simulink model "CalibrationMotorbike_v2"  (R2020b)
settings: Solver=FixedStepDiscrete  StartTime=0.0  StopTime=inf  FixedStep=0.01  RelTol=1e-3  EnableMultiTasking=on
undefined symbols (not defined in the file or in its folder): fdesignblkfcn, gcbh
libraries: dspstat3 x11, dsparch4 x3, simulink x2, dspswit3 x1
(part 1 of 2)
settings Model: DataDictionary=MOCA_DD.sldd  EnableAccessToBaseWorkspace=off  DataTypeOverride=Off  DataTypeOverrideAppliesTo=Floating-point  MinMaxOverflowLogging=ForceOff  SimulationMode=accelerator  OrderedModelArguments=off  Creator=stj1si  LastModifiedBy=HNA3SI
settings DataIOCC: SaveFormat=Array  SaveOutput=off  SignalLogging=off  SaveTime=off  ReturnWorkspaceOutputs=off
settings OptimizationCC: DefaultParameterBehavior=Inlined  DefaultUnderspecifiedDataType=single  InlineInvariantSignals=on  EnhancedBackFolding=on  CachingGlobalReferences=on  ExpressionDepthLimit=2147483647  NoFixptDivByZeroProtection=on  EfficientFloat2IntCast=on  LifeSpan=1  SimCompilerOptimization=on  EfficientTunableParamExpr=on
settings DebuggingCC: SolverPrmCheckMsg=warning  ParameterPrecisionLossMsg=none  AllowSymbolicDim=off  StateNameClashWarn=warning  SFUnexpectedBacktrackingDiag=warning  SFNoUnconditionalDefaultTransitionDiag=warning  SFExecutionAtInitializationDiag=none  ArithmeticOperatorsInVariantConditions=warning
settings HardwareCC: ProdBitPerPointer=32  ProdBitPerSizeT=32  ProdBitPerPtrDiffT=32  ProdLargestAtomicInteger=Long  ProdLargestAtomicFloat=Double  ProdEndianess=BigEndian  ProdWordSize=32  ProdHWDeviceType=Freescale->32-bit PowerPC
settings ModelReferenceCC: ModelReferenceNumInstancesAllowed=Single  PropagateSignalLabelsOutOfModel=off
settings SFSimCC: SimUseLocalCustomCode=off  MATLABDynamicMemAlloc=off  CustomCodeUndefinedFunction=UseInterfaceOnly
settings RTWCC: Description=Embedded Coder  SystemTargetFile=ert.tlc  GenCodeOnly=on  TemplateMakefile=ert_default_tmf  GenerateReport=on  RTWUseLocalCustomCode=off  IncludeHyperlinkInReport=on  LaunchReport=on  GenerateTraceInfo=on  GenerateTraceReport=on  GenerateTraceReportSl=on  GenerateTraceReportSf=on  GenerateTraceReportEml=on
settings CodeAppCC: IgnoreCustomStorageClasses=off  IgnoreTestpoints=on  CustomSymbolStrType=$N$R$M  CustomSymbolStrFcnArg=COCA_rt$I$N$M  CustomSymbolStrBlkIO=COCA_rtb_$N$M  StateflowObjectComments=on  InternalIdentifier=Classic
settings ERTTargetCC: TargetLangStandard=C99 (ISO)  MultiwordLength=2048  GenerateSampleERTMain=on  IncludeMdlTerminateFcn=off  CombineSignalStateStructs=on  SuppressErrorStatus=on  SupportNonFinite=off  SupportComplex=off  CastingMode=Standards  InlinedParameterPlacement=NonHierarchical  ERTSrcFileBannerTemplate=ert_code_template_ebike.cgt  ERTCustomFileTemplate=example_file_process.tlc  ERTFilePackagingFormat=Compact  PreserveExternInFcnDecls=off  SuppressUnreachableDefaultCases=off  EnableSignedLeftShifts=off  EnableSignedRightShifts=off  IndentStyle=Allman  EnableUserReplacementTypes=on
settings ConfigComp: CovEnable=on  CovScope=ReferencedModels  CovIncludeTopModel=off  CovMetricSettings=dw  CovHTMLOptions=-sRT=1 -sVT=0 -aTS=1 -bRG=1 -bTC=1 -hTR=0 -nFC=0 -nFD=1 -scm=1 -bcm=1 -xEv=0 -xEM=0  CovSaveCumulativeToWorkspaceVar=on  CovSaveSingleToWorkspaceVar=on  CovModelRefEnable=all  CovSFcnEnable=off

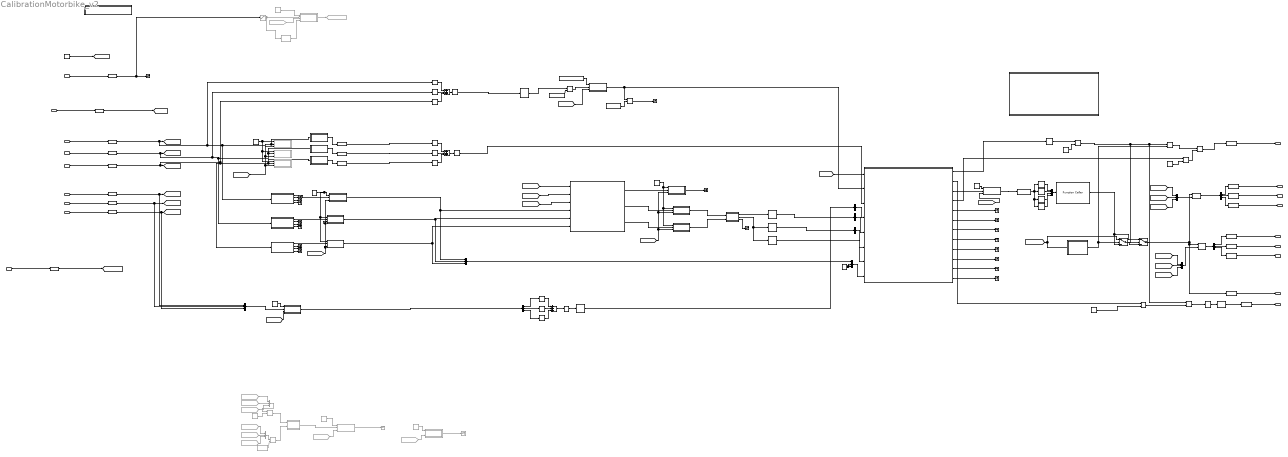
== system CalibrationMotorbike_v2 ==
  note: Detect, when rotMat has finished updating (falling edge)
  note: New: Bandpass instead Butterworth-Lowpass
      | Due to small differences (1g Offset) in diverse Smartphones a Bandpass is used, to remove noise and constant offset of Gravity
  note: if initRotMatrix availible and (current) Calibration not done use initRotMatrix for fast restart
      | (else use current intermediate rotmatrix or latest use current if calib done)
  note: Calibration done (passed all states)
  note: Curve Estimation (based on Gyro)
  note: Calculate Rotation Matrix from Gravity and Direction-angle
  note: Mounting of Smartphone in Driving-Direction (Extract Direction Angle)
  note: Strong Low-pass-Filtering to extract Gravity-Vector
  note: Test: IMU Fusion
  note: Test: IMU Fusion
  note: Variance of ACC-Rawdata as indication for Ignition/Engine ON and RIDING
  note: PreProcessing: 1st Level Lowpass Filtering
  note: Crop to Max
  note: X²+Y²+Z² drift in the 1g Offset during ride/engine on -> ignore this appoach
  note: Low-pass-Filtering to reduce HF-noise and disturbances (but still follow Bike-motion)
  note: Low-pass-Filtering to reduce HF-noise and disturbances (but still follow Bike-motion)
  note: Integration of Gyro-Signal to detect Curves etc.
      | Integration=Sum over Sliding Window (equals mean * windows-Size)
  note: Norm signal should be
      | =1g (=Gravity-Vector only) during standing/constant ride
      | !=1g when breaking/accelerating
  note: Continously Rotate Rawdata to current Gravity-direction
      | Attention: Gravity-Direction will be delayed (due to filtering) during motion compared to current rawdata
      | so output should only be used when gravity is almost constant
  note: 2nd Stage Filtering to further smoothen Signal
  note: should only contain Gravity = 1g
  note: Y/Z should contain Vector caused breaking/acceleration
      | (or 0 during constant riding)
  note: continously estimate driving-direction-angle
      | Warning: very noisy during constant ride or standing
      | (only stable direction during breaking/accelerating)
  note: 3rd Stage Filtering to even further smoothen Signal
      | Remark: driving direction angle might be very noisy
  note: Calibrate (Rotate) Rawdata
  note: Statemachine to estimate Driving/Situatin States
      | and extract Gravity&Direction-Vector for different Situations (Standing, Riding-Constant, Breaking)
  note: smoothen Calibration Vector to avoid Signal-jumps
  note: check for ignition
  "pressure [Pa] " : Inport
  accSfX [mg] : Inport  Port=2
  accSfY [mg] : Inport  Port=3
  accSfZ [mg] : Inport  Port=4
  gyrSfX [mdeg/s] : Inport  Port=5
  gyrSfY [mdeg/s] : Inport  Port=6
  gyrSfZ [mdeg/s] : Inport  Port=7
  speed [km/h*100]1 : Inport  Port=8
  initRotMatSf2Bf [3x3] : Inport  Port=9  PortDimensions=[3 3]
  Add : Sum  Inputs=+++
  Add1 : Sum  Inputs=+++
  Add2 : Sum  Inputs=+++
  Bandpass Filter3 : Subsystem  DialogController=fdesignblkfcn  InitFcn=fdesignblkfcn(gcbh, {'InitFcn'});  mask(Bandpass Filter){}
      mask help: Design a bandpass filter
      settings: CopyFcn=fdesignblkfcn(gcbh, {'CopyFcn'});
      mask Help: helpview(mapfilelocation('dsp'), 'dspbandpassfilter');
      mask Display: disp('Bandpass');
  Bandpass Filter4 : Subsystem  DialogController=fdesignblkfcn  InitFcn=fdesignblkfcn(gcbh, {'InitFcn'});  mask(Bandpass Filter){}
      mask help: Design a bandpass filter
      settings: CopyFcn=fdesignblkfcn(gcbh, {'CopyFcn'});
      mask Help: helpview(mapfilelocation('dsp'), 'dspbandpassfilter');
      mask Display: disp('Bandpass');
  Bandpass Filter5 : Subsystem  DialogController=fdesignblkfcn  InitFcn=fdesignblkfcn(gcbh, {'InitFcn'});  mask(Bandpass Filter){}
      mask help: Design a bandpass filter
      settings: CopyFcn=fdesignblkfcn(gcbh, {'CopyFcn'});
      mask Help: helpview(mapfilelocation('dsp'), 'dspbandpassfilter');
      mask Display: disp('Bandpass');
  Butterworth2nd1 : Subsystem  Commented=on
  Butterworth2nd10 : Subsystem
  Butterworth2nd11 : Subsystem
  Butterworth2nd12 : Subsystem
  Butterworth2nd13 : Subsystem
  Butterworth2nd14 : Subsystem  Commented=on
  Butterworth2nd16 : Subsystem
  Butterworth2nd2 : Subsystem  Commented=on
  Butterworth2nd3 : Subsystem  Commented=on
  Butterworth2nd4 : Subsystem  Commented=on
  Butterworth2nd5 : Subsystem
  Butterworth2nd6 : Subsystem
  Butterworth2nd7 : Subsystem  Commented=on
  Butterworth2nd8 : Subsystem
  Butterworth2nd9 : Subsystem
  CalibrationState : Stateflow chart  TreatAsAtomicUnit=on
  Cast To Single : DataTypeConversion  OutDataTypeStr=single
  Constant : Constant  Value=0.01
  Constant1 : Constant  Value=0.25
  Constant10 : Constant  Commented=on  Value=0.1
  Constant11 : Constant  Commented=on  Value=0.05
  Constant12 : Constant  Value=20000
  Constant13 : Constant  Value=0.25
  Constant14 : Constant  Value=0
  Constant15 : Constant  Value=4
  Constant16 : Constant  Value=0.1
  Constant17 : Constant
  Constant18 : Constant  Value=0
  Constant2 : Constant  Value=1000000
  Constant3 : Constant  Commented=on  Value=0.25
  Constant4 : Constant  Value=0.25
  Constant5 : Constant  Value=0.05
  Constant6 : Constant  Value=0.005
  Constant8 : Constant  Commented=on  Value=102
  Constant9 : Constant  Commented=on  Value=1000
  Data Type Conversion{1..3,5..9,11..12,14,24} (12 alike) : DataTypeConversion  OutDataTypeStr=single
  Data Type Conversion{10,13,15..19,23,27} (9 alike) : DataTypeConversion  RndMeth=Zero
  Demux : Demux  Outputs=3
  Demux1 : Demux  Outputs=1
  Demux2 : Demux  Outputs=1
  Demux3 : Demux  Outputs=3
  Demux4 : Demux  Outputs=1
  Demux5 : Demux  Outputs=3
  Direction_Vector : MATLAB Function  TreatAsAtomicUnit=on
  Divide : Product  Commented=on  Inputs=*/
  Divide1 : Product  Commented=on  Inputs=*/
  Double-Click Button to set current folder : Subsystem
      settings: OpenFcn=cd(fileparts(get_param(gcs,'filename')));
      mask Display: disp('\bf\fontsize{16}Double-Click to set current folder      ','texmode','on')
  Edge Detector : dspswit3/Edge Detector
      settings: SourceProductBaseCode=DS
  From15 : From  Commented=on  GotoTag=samplePeriod_s
  From31 : From  Commented=on  GotoTag=accSfXmg
  From32 : From  Commented=on  GotoTag=accSfYmg
  From33 : From  Commented=on  GotoTag=accSfZmg
  From34 : From  Commented=on  GotoTag=gyrSfXmdegs
  From35 : From  Commented=on  GotoTag=gyrSfYmdegs
  From36 : From  Commented=on  GotoTag=gyrSfZmdegs
  From37 : From  Commented=on  GotoTag=samplePeriod_s
  From9 : From  Commented=on  GotoTag=samplePeriod_s
  Function Caller : FunctionCaller  FunctionPrototype=rot_Matrix = Gravity_2_RotMatrix(gravity)  InputArgumentSpecifications=<Enter example>  OutputArgumentSpecifications=<Enter example>
  Goto69 : Goto  Commented=on  GotoTag=AtmPress_Filt
  GreaterThan : RelationalOperator  Operator=>  OutDataTypeStr=boolean  RndMeth=Simplest
  GreaterThanOrEqual : RelationalOperator  OutDataTypeStr=boolean  RndMeth=Simplest
  GreaterThanOrEqual1 : RelationalOperator  OutDataTypeStr=boolean  RndMeth=Simplest
  Logical Operator : Logic  AllPortsSameDT=off  OutDataTypeStr=boolean
  Logical Operator1 : Logic  Operator=OR  AllPortsSameDT=off  OutDataTypeStr=boolean
  Logical Operator2 : Logic  AllPortsSameDT=off  OutDataTypeStr=boolean
  MATLAB Function : MATLAB Function  Commented=on  TreatAsAtomicUnit=on
  MATLAB Function1 : MATLAB Function  TreatAsAtomicUnit=on
  Matrix Multiply : Product  Multiplication=Matrix(*)
  Matrix Multiply1 : Product  Multiplication=Matrix(*)
  Min1 : MinMax  Inputs=2
  Min2 : MinMax  Inputs=2
  Moving Average : dspstat3/Moving Average  Method=Sliding window  ForgettingFactorPort=off  SpecifyWindowLength=on  WindowLength=10  ForgettingFactor=0.9  SimulateUsing=Code generation
  Moving Average1 : dspstat3/Moving Average  Method=Sliding window  ForgettingFactorPort=off  SpecifyWindowLength=on  WindowLength=50  ForgettingFactor=0.9  SimulateUsing=Code generation
  Moving Average2 : dspstat3/Moving Average  Method=Sliding window  ForgettingFactorPort=off  SpecifyWindowLength=on  WindowLength=50  ForgettingFactor=0.9  SimulateUsing=Code generation
  Moving Variance2 : dspstat3/Moving Variance  Method=Sliding window  ForgettingFactorPort=off  SpecifyWindowLength=on  WindowLength=40  ForgettingFactor=0.9  SimulateUsing=Code generation
      settings: SourceProductBaseCode=DS
  Moving Variance4 : dspstat3/Moving Variance  Method=Sliding window  ForgettingFactorPort=off  SpecifyWindowLength=on  WindowLength=50  ForgettingFactor=0.9  SimulateUsing=Code generation
      settings: SourceProductBaseCode=DS
  Mux : Mux  Commented=on  Inputs=3
  Mux1 : Mux  Commented=on  Inputs=3
  Mux{2..6} (5 alike) : Mux  Inputs=3
  Mux7 : Mux
  NOT : Logic  Operator=NOT  AllPortsSameDT=off  OutDataTypeStr=boolean
  Rotate_to_Gravity : MATLAB Function  TreatAsAtomicUnit=on
  Saturation1 : Saturate  Commented=on  UpperLimit=120000  LowerLimit=80000
  Selector : Selector  InputPortWidth=12  IndexOptions=Index vector (dialog)  Indices=1  OutputSizes=1
  Selector1 : Selector  InputPortWidth=5  IndexOptions=Index vector (dialog)  Indices=1  OutputSizes=1
  Selector2 : Selector  InputPortWidth=5  IndexOptions=Index vector (dialog)  Indices=2  OutputSizes=1
  Selector3 : Selector  InputPortWidth=5  IndexOptions=Index vector (dialog)  Indices=3  OutputSizes=1
  Selector4 : Selector  InputPortWidth=5  IndexOptions=Index vector (dialog)  Indices=4  OutputSizes=1
  Simulink Function : Subsystem  TreatAsAtomicUnit=on
  SmartACCFilter1 : Subsystem
  SmartACCFilter2 : Subsystem
  SmartACCFilter3 : Subsystem
  Sqrt : Sqrt  SaturateOnIntegerOverflow=on
  Sqrt1 : Sqrt  SaturateOnIntegerOverflow=on
  Sqrt2 : Sqrt  SaturateOnIntegerOverflow=on
  Square{,1..8} (9 alike) : Math  Operator=square  SignedPower=on  SaturateOnIntegerOverflow=on
  Switch : Switch  Criteria=u2 > Threshold
  Switch1 : Switch  Criteria=u2 > Threshold
  Terminator{,1..18,21..22} (21 alike) : Terminator
  Terminator19 : Terminator  Commented=on
  Terminator20 : Terminator  Commented=on
  Transfer Fcn First Order2 : simulink/Discrete/Transfer Fcn First Order  Commented=on  PoleZ=0.95  ICPrevOutput=90000  DoSatur=off
  accBfX [mg] : Outport  VectorParamsAs1DForOutWhenUnconnected=off
  accBfY [mg] : Outport  Port=2  VectorParamsAs1DForOutWhenUnconnected=off
  accBfZ [mg] : Outport  Port=3  VectorParamsAs1DForOutWhenUnconnected=off
  gyrBfX [mdeg/s] : Outport  Port=4  VectorParamsAs1DForOutWhenUnconnected=off
  gyrBfY [mdeg/s] : Outport  Port=5  VectorParamsAs1DForOutWhenUnconnected=off
  gyrBfZ [mdeg/s] : Outport  Port=6  VectorParamsAs1DForOutWhenUnconnected=off
  calibFlag [0/1] : Outport  Port=7  VectorParamsAs1DForOutWhenUnconnected=off
  rotMatSf2Bf [3x3] : Outport  Port=8  VectorParamsAs1DForOutWhenUnconnected=off
  rotMatUpdate [0/1] : Outport  Port=9  VectorParamsAs1DForOutWhenUnconnected=off
  wires:
  accSfY [mg]/1 -> Data Type Conversion3/1  "ACC_accSfYmg"
  accSfX [mg]/1 -> Data Type Conversion2/1  "ACC_accSfXmg"
  "pressure [Pa] "/1 -> Data Type Conversion12/1  "ENV_pressurePa"
  accSfZ [mg]/1 -> Data Type Conversion1/1  "ACC_accSfZmg"
  gyrSfX [mdeg/s]/1 -> Data Type Conversion8/1  "GYR_gyrSfXmdegs"
  gyrSfY [mdeg/s]/1 -> Data Type Conversion9/1  "GYR_gyrSfYmdegs"
  gyrSfZ [mdeg/s]/1 -> Data Type Conversion7/1  "GYR_gyrSfZmdegs"
  Data Type Conversion10/1 -> accBfX [mg]/1  "COCA_accBfXmg"
  Data Type Conversion13/1 -> accBfY [mg]/1  "COCA_accBfYmg"
  Data Type Conversion15/1 -> accBfZ [mg]/1  "COCA_accBfZmg"
  Data Type Conversion16/1 -> gyrBfX [mdeg/s]/1  "COCA_gyrBfXmdegs"
  Data Type Conversion17/1 -> gyrBfY [mdeg/s]/1  "COCA_gyrBfYmdegs"
  Data Type Conversion18/1 -> gyrBfZ [mdeg/s]/1  "COCA_gyrBfZmdegs"
  Data Type Conversion12/1 -> Saturation1/1, Terminator22/1  "pressure_Pa"
  Data Type Conversion8/1 -> Mux2/1, [gyrSfXmdegs]  "gyrSfX_mdegs"
  Data Type Conversion9/1 -> Mux2/2, [gyrSfYmdegs]  "gyrSfY_mdegs"
  Data Type Conversion7/1 -> Mux2/3, [gyrSfZmdegs]  "gyrSfZ_mdegs"
  Constant11/1 -> Butterworth2nd4/1(cutOff-Freq)
  From15/1 -> Butterworth2nd4/3(samplingTime)
  Butterworth2nd4/1(Y(t)) -> Goto69/1  "AtmPressureFilt"
  Constant/1 -> [samplePeriod_s]
  Demux5/1 -> Data Type Conversion16/1
  Demux5/2 -> Data Type Conversion17/1
  Demux5/3 -> Data Type Conversion18/1
  Transfer Fcn First Order2/1 -> Butterworth2nd4/4(prefilteredVal)  "AtmPressureFiltTransFer"
  Data Type Conversion19/1 -> calibFlag [0/1]/1  "COCA_calibrationFlag"
  Saturation1/1 -> Butterworth2nd4/2(U(t)), Transfer Fcn First Order2/1
  Data Type Conversion2/1 -> SmartACCFilter2/1(ACC_In), Bandpass Filter3/1(In), Butterworth2nd1/2(U(t)), Square3/1, [accSfXmg]  "accSfX_mg"
  Data Type Conversion3/1 -> Square4/1, SmartACCFilter1/1(ACC_In), Bandpass Filter4/1(In), Butterworth2nd2/2(U(t)), [accSfYmg]  "accSfY_mg"
  Data Type Conversion1/1 -> Square5/1, SmartACCFilter3/1(ACC_In), Bandpass Filter5/1(In), Butterworth2nd3/2(U(t)), [accSfZmg]  "accSfZ_mg"
  Add/1 -> Sqrt/1
  Square2/1 -> Add/3
  Square/1 -> Add/1
  Square1/1 -> Add/2
  Data Type Conversion11/1 -> Square2/1
  Data Type Conversion6/1 -> Square1/1
  Data Type Conversion5/1 -> Square/1
  Bandpass Filter5/1(Out) -> Data Type Conversion11/1  "accSfZFilt_mg"
  Bandpass Filter4/1(Out) -> Data Type Conversion6/1  "accSfYFilt_mg"
  Bandpass Filter3/1(Out) -> Data Type Conversion5/1  "accSfXFilt_mg"
  Constant1/1 -> Butterworth2nd1/1(cutOff-Freq), Butterworth2nd2/1(cutOff-Freq), Butterworth2nd3/1(cutOff-Freq)
  [samplePeriod_s] -> Butterworth2nd3/3(samplingTime), Butterworth2nd2/3(samplingTime), Butterworth2nd1/3(samplingTime)
  Square4/1 -> Add1/2
  Square3/1 -> Add1/1
  Square5/1 -> Add1/3
  Constant2/1 -> Min1/2
  Constant5/1 -> Butterworth2nd6/1(cutOff-Freq)
  Min1/1 -> Butterworth2nd6/2(U(t))
  [samplePeriod_s] -> Butterworth2nd6/3(samplingTime)
  Butterworth2nd6/1(Y(t)) -> Min2/1, CalibrationState/2(accSfmg_Variance)  "accSfmg_Variance_filt"
  Moving Variance2/1 -> Min1/1  "accSfmg_ABSvariance40"
  Add1/1 -> Sqrt1/1
  Sqrt1/1 -> Moving Variance2/1  "accSfNorm_Raw"
  From9/1 -> Butterworth2nd7/3(samplingTime)
  Constant3/1 -> Butterworth2nd7/1(cutOff-Freq)
  Butterworth2nd7/1(Y(t)) -> Terminator20/1  "accSfNorm_Filt"
  [accSfXmg] -> Rotate_to_Gravity/1(x)
  [accSfYmg] -> Rotate_to_Gravity/2(y)
  [accSfZmg] -> Rotate_to_Gravity/3(z)
  Rotate_to_Gravity/1(x_rot) -> Butterworth2nd8/2(U(t))  "accSfXmg_rot"
  Rotate_to_Gravity/2(y_rot) -> Butterworth2nd9/2(U(t))  "accSfYmg_rot"
  Rotate_to_Gravity/3(z_rot) -> Butterworth2nd10/2(U(t))  "accSfZmg_rot"
  Constant4/1 -> Butterworth2nd10/1(cutOff-Freq), Butterworth2nd9/1(cutOff-Freq), Butterworth2nd8/1(cutOff-Freq)
  [samplePeriod_s] -> Butterworth2nd10/3(samplingTime), Butterworth2nd9/3(samplingTime), Butterworth2nd8/3(samplingTime)
  Butterworth2nd8/1(Y(t)) -> Terminator18/1  "accSfXmg_rotFilt"
  Butterworth2nd9/1(Y(t)) -> Direction_Vector/1(y)  "accSfYmg_rotFilt"
  Butterworth2nd10/1(Y(t)) -> Direction_Vector/2(z)  "accSfZmg_rotFilt"
  Direction_Vector/1(abs) -> Moving Average1/1  "Direction_abs"
  Direction_Vector/2(alpha) -> Moving Average2/1, Moving Variance4/1  "Direction_alpha"
  Constant6/1 -> Butterworth2nd11/1(cutOff-Freq), Butterworth2nd12/1(cutOff-Freq), Butterworth2nd13/1(cutOff-Freq)
  [samplePeriod_s] -> Butterworth2nd13/3(samplingTime), Butterworth2nd12/3(samplingTime), Butterworth2nd11/3(samplingTime)
  Butterworth2nd11/1(Y(t)) -> Rotate_to_Gravity/4(x_gravity), Mux3/1  "accSfXmg_SmartFilt"
  Butterworth2nd12/1(Y(t)) -> Rotate_to_Gravity/5(y_gravity), Mux3/2  "accSfYmg_SmartFilt"
  Butterworth2nd13/1(Y(t)) -> Rotate_to_Gravity/6(z_gravity), Mux3/3  "accSfZmg_SmartFilt"
  SmartACCFilter3/1(accSf_mg_SmartFilter) -> Butterworth2nd13/2(U(t))  "accSfZmg_Smart"
  SmartACCFilter1/1(accSf_mg_SmartFilter) -> Butterworth2nd12/2(U(t))  "accSfYmg_Smart"
  SmartACCFilter2/1(accSf_mg_SmartFilter) -> Butterworth2nd11/2(U(t))  "accSfXmg_Smart"
  From31/1 -> Mux/1
  From32/1 -> Mux/2
  From33/1 -> Mux/3
  From34/1 -> Mux1/1
  From35/1 -> Mux1/2
  From36/1 -> Mux1/3
  Mux/1 -> Divide/1
  Divide/1 -> MATLAB Function/1(accel)
  Constant8/1 -> Divide/2
  Mux1/1 -> Divide1/1
  Divide1/1 -> MATLAB Function/2(gyro)
  Constant9/1 -> Divide1/2
  Constant10/1 -> Butterworth2nd14/1(cutOff-Freq)
  From37/1 -> Butterworth2nd14/3(samplingTime)
  Butterworth2nd14/1(Y(t)) -> Terminator19/1  "accel_RotFilt"
  MATLAB Function/1(accel_rot) -> Butterworth2nd14/2(U(t))  "accel_Rot"
  Mux3/1 -> Mux4/1  "accSfYmg_Gravity"
  [samplePeriod_s] -> Butterworth2nd16/3(samplingTime)
  Constant13/1 -> Butterworth2nd16/1(cutOff-Freq)
  Mux2/1 -> Butterworth2nd16/2(U(t))
  Moving Average/1 -> Demux4/1  "gyrSfmdegs_FiltAverage"
  Demux/1 -> Square6/1
  Demux/2 -> Square7/1
  Demux/3 -> Square8/1
  Square7/1 -> Add2/2
  Square6/1 -> Add2/1
  Square8/1 -> Add2/3
  Add2/1 -> Sqrt2/1
  Butterworth2nd16/1(Y(t)) -> Demux/1  "gyrSfmdegs_Filt"
  Sqrt2/1 -> Moving Average/1
  CalibrationState/5(state_Riding) -> Terminator9/1  "state_Riding"
  CalibrationState/4(state_Ignition) -> GreaterThanOrEqual1/1  "state_Ignition"
  CalibrationState/6(state_Acceleration) -> Terminator10/1  "state_Acceleration"
  CalibrationState/7(state_Curve) -> Terminator11/1  "state_Curve"
  CalibrationState/2(state_Calibration) -> GreaterThan/1  "state_Calibration"
  CalibrationState/8(state_Direction) -> Terminator12/1  "state_Direction"
  Moving Average1/1 -> Demux1/1  "Direction_absAverage"
  Demux1/1 -> CalibrationState/5(Direction_absAverage)
  Moving Average2/1 -> CalibrationState/7(Direction_alpha)  "Direction_alphaAverage"
  Moving Variance4/1 -> Demux2/1  "Direction_alpha_Variance"
  Demux2/1 -> CalibrationState/6(Direction_alpha_Variance)
  Demux4/1 -> CalibrationState/4(gyrSfmdegs_FiltAverage)
  CalibrationState/9(GravityStanding) -> Terminator13/1  "GravityStanding"
  CalibrationState/10(GravityRiding) -> Terminator14/1  "GravityRiding"
  CalibrationState/11(GravityBreaking) -> Terminator15/1  "GravityBreaking"
  Constant14/1 -> Mux4/2, Mux4/3
  Mux4/1 -> CalibrationState/8(Gravity)
  [accSfXmg] -> Mux5/1
  [accSfYmg] -> Mux5/2
  [accSfZmg] -> Mux5/3
  [gyrSfZmdegs] -> Mux6/3
  [gyrSfYmdegs] -> Mux6/2
  [gyrSfXmdegs] -> Mux6/1
  Matrix Multiply1/1 -> Demux5/1  "gyrBfmdegs"
  Constant15/1 -> GreaterThanOrEqual/2
  Selector/1 -> GreaterThanOrEqual/1
  CalibrationState/1(calibrationOUT) -> Selector/1  "calibration"
  Demux3/1 -> Data Type Conversion10/1
  Demux3/2 -> Data Type Conversion13/1
  Demux3/3 -> Data Type Conversion15/1
  Mux6/1 -> Matrix Multiply1/2
  Mux5/1 -> Matrix Multiply/2
  Selector1/1 -> Mux7/1
  Selector2/1 -> Mux7/2
  Selector3/1 -> Mux7/3
  Cast To Single/1 -> Selector1/1, Selector2/1, Selector4/1, Selector3/1
  Selector4/1 -> Mux7/4
  Function Caller/1 -> Switch1/1, Switch/3  "rot_Matrix"
  Matrix Multiply/1 -> Demux3/1  "accBfmg"
  Direction_Vector/3(alphastate) -> Terminator17/1  "Direction_alphaState"
  Constant12/1 -> Min2/2
  Min2/1 -> Terminator21/1  "accSfmg_Variance_filt_cropped"
  Sqrt/1 -> CalibrationState/3(accFiltSfNorm)  "accFiltNorm"
  CalibrationState/12(GravityAccel) -> Terminator16/1  "GravityAccel"
  Constant16/1 -> Butterworth2nd5/1(cutOff-Freq)
  [samplePeriod_s] -> Butterworth2nd5/3(samplingTime)
  Butterworth2nd5/1(Y(t)) -> Cast To Single/1  "Calibration_Vector_Filt"
  Mux7/1 -> Function Caller/1
  CalibrationState/3(Calibration_Vector) -> Butterworth2nd5/2(U(t))  "Calibration_Vector"
  Constant17/1 -> GreaterThanOrEqual1/2
  GreaterThanOrEqual/1 -> Switch1/2, Logical Operator2/1, Logical Operator1/1
  GreaterThanOrEqual1/1 -> Logical Operator/2  "calibFlag"
  Logical Operator/1 -> Data Type Conversion19/1  "calibFlag"
  Data Type Conversion27/1 -> rotMatUpdate [0/1]/1  "rotMatUpdate"
  Data Type Conversion23/1 -> rotMatSf2Bf [3x3]/1  "rotMatSf2BfOut_3x3"
  Constant18/1 -> GreaterThan/2
  initRotMatSf2Bf [3x3]/1 -> Data Type Conversion24/1  "initRotMatSf2Bf_3x3"
  speed [km/h*100]1/1 -> Data Type Conversion14/1  "SPECO_getPresentSpeed"
  Data Type Conversion14/1 -> [speed_kmh]  "speedKmh"
  Data Type Conversion24/1 -> [initRotMat]
  [speed_kmh] -> CalibrationState/1(speed_kmh)
  [initRotMat] -> Switch/1, MATLAB Function1/1(initRotMat)
  MATLAB Function1/1(init_valid) -> Logical Operator1/2, Switch/2
  Switch/1 -> Switch1/3
  Switch1/1 -> Matrix Multiply/1, Data Type Conversion23/1, Matrix Multiply1/1
  Logical Operator1/1 -> Logical Operator/1
  SmartACCFilter2/2(accSf_mg_SmartFilter_k) -> Terminator/1
  SmartACCFilter2/3(accSf_mg_Average20) -> Terminator1/1  "accSfXmg_Average"
  SmartACCFilter2/4(accSf_mg_Std20) -> Terminator2/1
  SmartACCFilter1/2(accSf_mg_SmartFilter_k) -> Terminator3/1
  SmartACCFilter1/3(accSf_mg_Average20) -> Terminator4/1  "accSfYmg_Average"
  SmartACCFilter1/4(accSf_mg_Std20) -> Terminator5/1
  SmartACCFilter3/2(accSf_mg_SmartFilter_k) -> Terminator6/1
  SmartACCFilter3/3(accSf_mg_Average20) -> Terminator7/1  "accSfZmg_Average"
  SmartACCFilter3/4(accSf_mg_Std20) -> Terminator8/1
  GreaterThan/1 -> Logical Operator2/2
  Logical Operator2/1 -> NOT/1
  NOT/1 -> Edge Detector/1
  Edge Detector/1 -> Data Type Conversion27/1

== system CalibrationMotorbike_v2/Bandpass Filter3 ==
  In : Inport
  Generated Filter Block : dsparch4/Biquad Filter  Tag=BlockMethodSubSystem  FilterSource=Dialog parameters  CoeffSource=Specify via dialog  FilterObject=BQF  IIRFiltStruct=Direct form II  BiQuadCoeffs=[2 0 -2 1 -1.99938112988008743 0.999381493758366379;2 0 -2 1 -1.9520719762606884 0.954121525383550995]  ScaleValues=[3.21383336440108381e-07;1;350.750828850398136]  IC=0  ICnum=0  ICden=0  a0Flag=Warning  optimizeScaleValues=off  ScaleValueMode=Specify via input port (g)  InputProcessing=Columns as channels (frame based)  roundingMode=Floor  overflowMode=off  scaleValueFracLength=14  denProdOutputFracLength=30  denAccumFracLength=30  secondMemoryFracLength=15
  Out : Outport  VectorParamsAs1DForOutWhenUnconnected=off
  wires:
  In/1 -> Generated Filter Block/1
  Generated Filter Block/1 -> Out/1

== system CalibrationMotorbike_v2/Bandpass Filter4 ==
  In : Inport
  Generated Filter Block : dsparch4/Biquad Filter  Tag=BlockMethodSubSystem  FilterSource=Dialog parameters  CoeffSource=Specify via dialog  FilterObject=BQF  IIRFiltStruct=Direct form II  BiQuadCoeffs=[2 0 -2 1 -1.99938112988008743 0.999381493758366379;2 0 -2 1 -1.9520719762606884 0.954121525383550995]  ScaleValues=[3.21383336440108381e-07;1;350.750828850398136]  IC=0  ICnum=0  ICden=0  a0Flag=Warning  optimizeScaleValues=off  ScaleValueMode=Specify via input port (g)  InputProcessing=Columns as channels (frame based)  roundingMode=Floor  overflowMode=off  scaleValueFracLength=14  denProdOutputFracLength=30  denAccumFracLength=30  secondMemoryFracLength=15
  Out : Outport  VectorParamsAs1DForOutWhenUnconnected=off
  wires:
  Generated Filter Block/1 -> Out/1
  In/1 -> Generated Filter Block/1

== system CalibrationMotorbike_v2/Bandpass Filter5 ==
  In : Inport
  Generated Filter Block : dsparch4/Biquad Filter  Tag=BlockMethodSubSystem  FilterSource=Dialog parameters  CoeffSource=Specify via dialog  FilterObject=BQF  IIRFiltStruct=Direct form II  BiQuadCoeffs=[2 0 -2 1 -1.99938112988008743 0.999381493758366379;2 0 -2 1 -1.9520719762606884 0.954121525383550995]  ScaleValues=[3.21383336440108381e-07;1;350.750828850398136]  IC=0  ICnum=0  ICden=0  a0Flag=Warning  optimizeScaleValues=off  ScaleValueMode=Specify via input port (g)  InputProcessing=Columns as channels (frame based)  roundingMode=Floor  overflowMode=off  scaleValueFracLength=14  denProdOutputFracLength=30  denAccumFracLength=30  secondMemoryFracLength=15
  Out : Outport  VectorParamsAs1DForOutWhenUnconnected=off
  wires:
  Generated Filter Block/1 -> Out/1
  In/1 -> Generated Filter Block/1

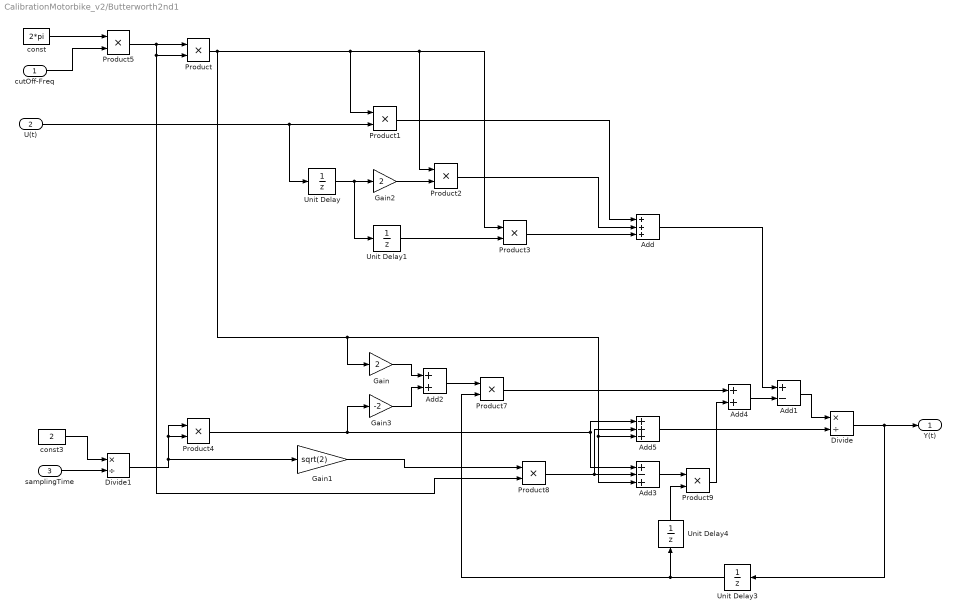
== system CalibrationMotorbike_v2/Butterworth2nd1 ==
  cutOff-Freq : Inport
  U(t) : Inport  Port=2
  samplingTime : Inport  Port=3
  Add : Sum  Inputs=+++
  Add1 : Sum  Inputs=+-
  Add2 : Sum
  Add3 : Sum  Inputs=+-+
  Add4 : Sum
  Add5 : Sum  Inputs=+++
  Divide : Product  Inputs=*/
  Divide1 : Product  Inputs=*/
  Gain : Gain  Gain=2
  Gain1 : Gain  Gain=sqrt(2)
  Gain2 : Gain  Gain=2
  Gain3 : Gain  Gain=-2
  Product{,1..5,7..9} (9 alike) : Product  RndMeth=Zero
  Unit Delay{,1,3..4} (4 alike) : UnitDelay  SampleTime=-1  HasFrameUpgradeWarning=on
  const : Constant  Value=2*pi
  const3 : Constant  Value=2
  Y(t) : Outport  VectorParamsAs1DForOutWhenUnconnected=off
  wires:
  U(t)/1 -> Product1/2, Unit Delay/1
  Product/1 -> Product1/1, Product3/1, Product2/1, Gain/1, Add3/3, Add5/3
  Unit Delay/1 -> Unit Delay1/1, Gain2/1
  Unit Delay1/1 -> Product3/2
  Product1/1 -> Add/1
  Product2/1 -> Add/2
  Product3/1 -> Add/3
  Add/1 -> Add1/1
  Divide/1 -> Unit Delay3/1, Y(t)/1
  Product4/1 -> Add3/1, Add5/1, Gain3/1
  Gain/1 -> Add2/1
  Unit Delay3/1 -> Product7/2, Unit Delay4/1
  Add2/1 -> Product7/1
  Gain1/1 -> Product8/1
  Product8/1 -> Add3/2, Add5/2
  Unit Delay4/1 -> Product9/2
  Add3/1 -> Product9/1
  Product9/1 -> Add4/2
  Product7/1 -> Add4/1
  Add4/1 -> Add1/2
  Add1/1 -> Divide/1
  Add5/1 -> Divide/2
  Gain2/1 -> Product2/2
  Gain3/1 -> Add2/2
  Product5/1 -> Product/1, Product/2, Product8/2
  const/1 -> Product5/1
  cutOff-Freq/1 -> Product5/2
  const3/1 -> Divide1/1
  samplingTime/1 -> Divide1/2
  Divide1/1 -> Gain1/1, Product4/2, Product4/1

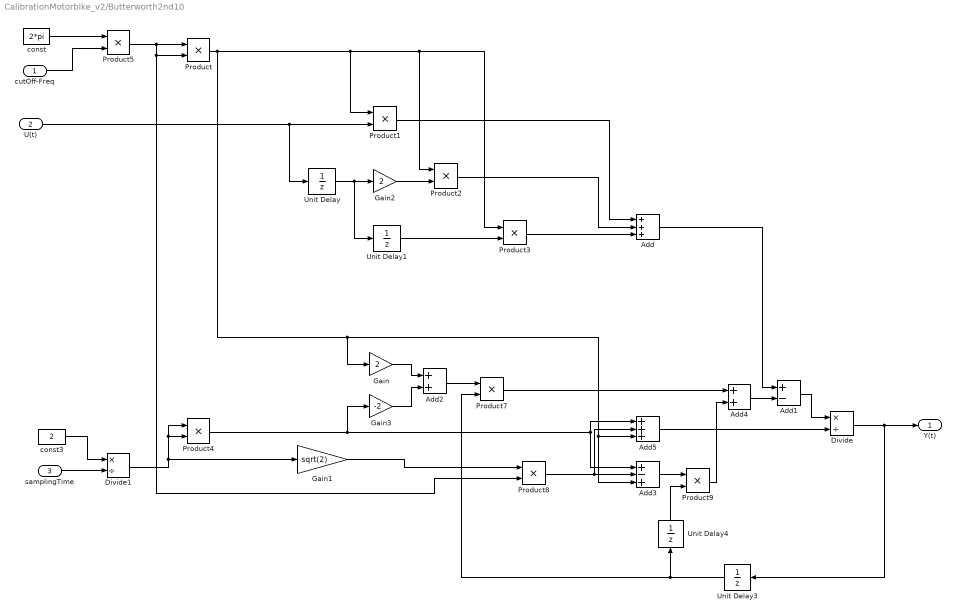
== system CalibrationMotorbike_v2/Butterworth2nd10 ==
  cutOff-Freq : Inport
  U(t) : Inport  Port=2
  samplingTime : Inport  Port=3
  Add : Sum  Inputs=+++
  Add1 : Sum  Inputs=+-
  Add2 : Sum
  Add3 : Sum  Inputs=+-+
  Add4 : Sum
  Add5 : Sum  Inputs=+++
  Divide : Product  Inputs=*/
  Divide1 : Product  Inputs=*/
  Gain : Gain  Gain=2
  Gain1 : Gain  Gain=sqrt(2)
  Gain2 : Gain  Gain=2
  Gain3 : Gain  Gain=-2
  Product{,1..5,7..9} (9 alike) : Product  RndMeth=Zero
  Unit Delay{,1,3..4} (4 alike) : UnitDelay  SampleTime=-1  HasFrameUpgradeWarning=on
  const : Constant  Value=2*pi
  const3 : Constant  Value=2
  Y(t) : Outport  VectorParamsAs1DForOutWhenUnconnected=off
  wires:
  Divide1/1 -> Product4/1, Product4/2, Gain1/1
  samplingTime/1 -> Divide1/2
  const3/1 -> Divide1/1
  cutOff-Freq/1 -> Product5/2
  const/1 -> Product5/1
  Product5/1 -> Product8/2, Product/2, Product/1
  Gain3/1 -> Add2/2
  Gain2/1 -> Product2/2
  Add5/1 -> Divide/2
  Add1/1 -> Divide/1
  Add4/1 -> Add1/2
  Product7/1 -> Add4/1
  Product9/1 -> Add4/2
  Add3/1 -> Product9/1
  Unit Delay4/1 -> Product9/2
  Product8/1 -> Add5/2, Add3/2
  Gain1/1 -> Product8/1
  Add2/1 -> Product7/1
  Unit Delay3/1 -> Unit Delay4/1, Product7/2
  Gain/1 -> Add2/1
  Product4/1 -> Gain3/1, Add5/1, Add3/1
  Divide/1 -> Y(t)/1, Unit Delay3/1
  Add/1 -> Add1/1
  Product3/1 -> Add/3
  Product2/1 -> Add/2
  Product1/1 -> Add/1
  Unit Delay1/1 -> Product3/2
  Unit Delay/1 -> Gain2/1, Unit Delay1/1
  Product/1 -> Add5/3, Add3/3, Gain/1, Product2/1, Product3/1, Product1/1
  U(t)/1 -> Unit Delay/1, Product1/2

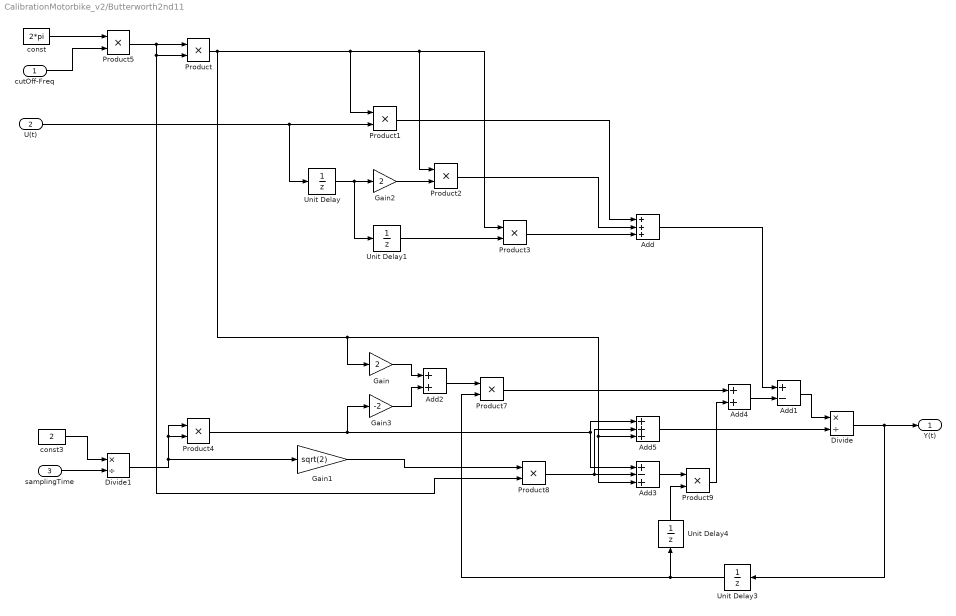
== system CalibrationMotorbike_v2/Butterworth2nd11 ==
  cutOff-Freq : Inport
  U(t) : Inport  Port=2
  samplingTime : Inport  Port=3
  Add : Sum  Inputs=+++
  Add1 : Sum  Inputs=+-
  Add2 : Sum
  Add3 : Sum  Inputs=+-+
  Add4 : Sum
  Add5 : Sum  Inputs=+++
  Divide : Product  Inputs=*/
  Divide1 : Product  Inputs=*/
  Gain : Gain  Gain=2
  Gain1 : Gain  Gain=sqrt(2)
  Gain2 : Gain  Gain=2
  Gain3 : Gain  Gain=-2
  Product{,1..5,7..9} (9 alike) : Product  RndMeth=Zero
  Unit Delay{,1,3..4} (4 alike) : UnitDelay  SampleTime=-1  HasFrameUpgradeWarning=on
  const : Constant  Value=2*pi
  const3 : Constant  Value=2
  Y(t) : Outport  VectorParamsAs1DForOutWhenUnconnected=off
  wires:
  Divide1/1 -> Product4/1, Product4/2, Gain1/1
  samplingTime/1 -> Divide1/2
  const3/1 -> Divide1/1
  cutOff-Freq/1 -> Product5/2
  const/1 -> Product5/1
  Product5/1 -> Product8/2, Product/2, Product/1
  Gain3/1 -> Add2/2
  Gain2/1 -> Product2/2
  Add5/1 -> Divide/2
  Add1/1 -> Divide/1
  Add4/1 -> Add1/2
  Product7/1 -> Add4/1
  Product9/1 -> Add4/2
  Add3/1 -> Product9/1
  Unit Delay4/1 -> Product9/2
  Product8/1 -> Add5/2, Add3/2
  Gain1/1 -> Product8/1
  Add2/1 -> Product7/1
  Unit Delay3/1 -> Unit Delay4/1, Product7/2
  Gain/1 -> Add2/1
  Product4/1 -> Gain3/1, Add5/1, Add3/1
  Divide/1 -> Y(t)/1, Unit Delay3/1
  Add/1 -> Add1/1
  Product3/1 -> Add/3
  Product2/1 -> Add/2
  Product1/1 -> Add/1
  Unit Delay1/1 -> Product3/2
  Unit Delay/1 -> Gain2/1, Unit Delay1/1
  Product/1 -> Add5/3, Add3/3, Gain/1, Product2/1, Product3/1, Product1/1
  U(t)/1 -> Unit Delay/1, Product1/2

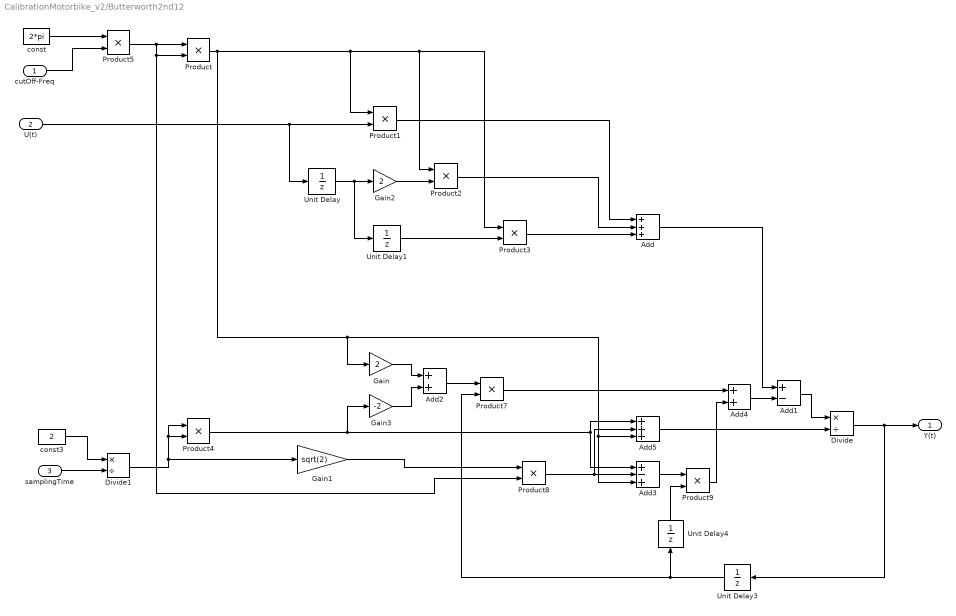
== system CalibrationMotorbike_v2/Butterworth2nd12 ==
  cutOff-Freq : Inport
  U(t) : Inport  Port=2
  samplingTime : Inport  Port=3
  Add : Sum  Inputs=+++
  Add1 : Sum  Inputs=+-
  Add2 : Sum
  Add3 : Sum  Inputs=+-+
  Add4 : Sum
  Add5 : Sum  Inputs=+++
  Divide : Product  Inputs=*/
  Divide1 : Product  Inputs=*/
  Gain : Gain  Gain=2
  Gain1 : Gain  Gain=sqrt(2)
  Gain2 : Gain  Gain=2
  Gain3 : Gain  Gain=-2
  Product{,1..5,7..9} (9 alike) : Product  RndMeth=Zero
  Unit Delay{,1,3..4} (4 alike) : UnitDelay  SampleTime=-1  HasFrameUpgradeWarning=on
  const : Constant  Value=2*pi
  const3 : Constant  Value=2
  Y(t) : Outport  VectorParamsAs1DForOutWhenUnconnected=off
  wires:
  U(t)/1 -> Product1/2, Unit Delay/1
  Product/1 -> Product1/1, Product3/1, Product2/1, Gain/1, Add3/3, Add5/3
  Unit Delay/1 -> Unit Delay1/1, Gain2/1
  Unit Delay1/1 -> Product3/2
  Product1/1 -> Add/1
  Product2/1 -> Add/2
  Product3/1 -> Add/3
  Add/1 -> Add1/1
  Divide/1 -> Unit Delay3/1, Y(t)/1
  Product4/1 -> Add3/1, Add5/1, Gain3/1
  Gain/1 -> Add2/1
  Unit Delay3/1 -> Product7/2, Unit Delay4/1
  Add2/1 -> Product7/1
  Gain1/1 -> Product8/1
  Product8/1 -> Add3/2, Add5/2
  Unit Delay4/1 -> Product9/2
  Add3/1 -> Product9/1
  Product9/1 -> Add4/2
  Product7/1 -> Add4/1
  Add4/1 -> Add1/2
  Add1/1 -> Divide/1
  Add5/1 -> Divide/2
  Gain2/1 -> Product2/2
  Gain3/1 -> Add2/2
  Product5/1 -> Product/1, Product/2, Product8/2
  const/1 -> Product5/1
  cutOff-Freq/1 -> Product5/2
  const3/1 -> Divide1/1
  samplingTime/1 -> Divide1/2
  Divide1/1 -> Gain1/1, Product4/2, Product4/1

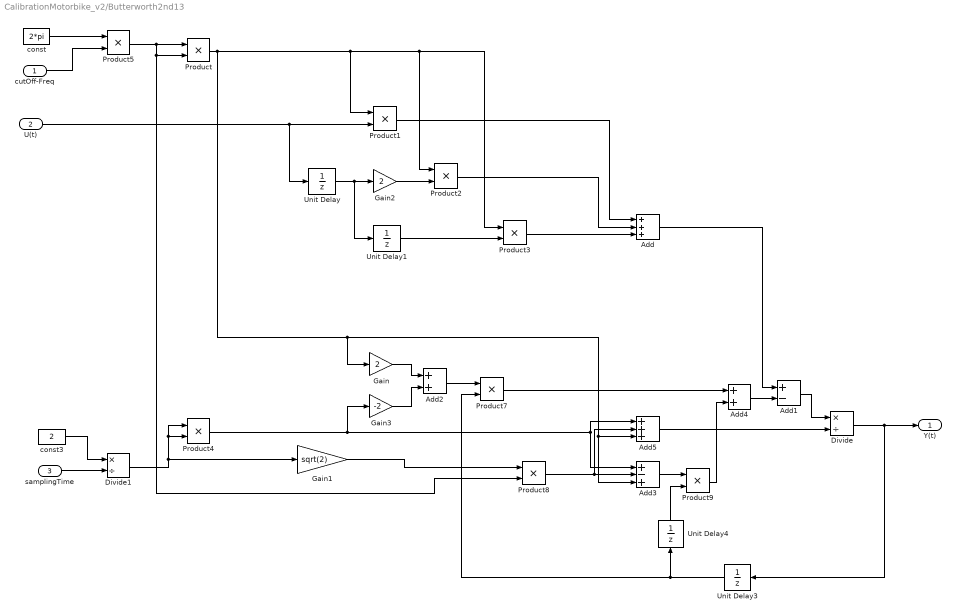
== system CalibrationMotorbike_v2/Butterworth2nd13 ==
  cutOff-Freq : Inport
  U(t) : Inport  Port=2
  samplingTime : Inport  Port=3
  Add : Sum  Inputs=+++
  Add1 : Sum  Inputs=+-
  Add2 : Sum
  Add3 : Sum  Inputs=+-+
  Add4 : Sum
  Add5 : Sum  Inputs=+++
  Divide : Product  Inputs=*/
  Divide1 : Product  Inputs=*/
  Gain : Gain  Gain=2
  Gain1 : Gain  Gain=sqrt(2)
  Gain2 : Gain  Gain=2
  Gain3 : Gain  Gain=-2
  Product{,1..5,7..9} (9 alike) : Product  RndMeth=Zero
  Unit Delay{,1,3..4} (4 alike) : UnitDelay  SampleTime=-1  HasFrameUpgradeWarning=on
  const : Constant  Value=2*pi
  const3 : Constant  Value=2
  Y(t) : Outport  VectorParamsAs1DForOutWhenUnconnected=off
  wires:
  Divide1/1 -> Product4/1, Product4/2, Gain1/1
  samplingTime/1 -> Divide1/2
  const3/1 -> Divide1/1
  cutOff-Freq/1 -> Product5/2
  const/1 -> Product5/1
  Product5/1 -> Product8/2, Product/2, Product/1
  Gain3/1 -> Add2/2
  Gain2/1 -> Product2/2
  Add5/1 -> Divide/2
  Add1/1 -> Divide/1
  Add4/1 -> Add1/2
  Product7/1 -> Add4/1
  Product9/1 -> Add4/2
  Add3/1 -> Product9/1
  Unit Delay4/1 -> Product9/2
  Product8/1 -> Add5/2, Add3/2
  Gain1/1 -> Product8/1
  Add2/1 -> Product7/1
  Unit Delay3/1 -> Unit Delay4/1, Product7/2
  Gain/1 -> Add2/1
  Product4/1 -> Gain3/1, Add5/1, Add3/1
  Divide/1 -> Y(t)/1, Unit Delay3/1
  Add/1 -> Add1/1
  Product3/1 -> Add/3
  Product2/1 -> Add/2
  Product1/1 -> Add/1
  Unit Delay1/1 -> Product3/2
  Unit Delay/1 -> Gain2/1, Unit Delay1/1
  Product/1 -> Add5/3, Add3/3, Gain/1, Product2/1, Product3/1, Product1/1
  U(t)/1 -> Unit Delay/1, Product1/2

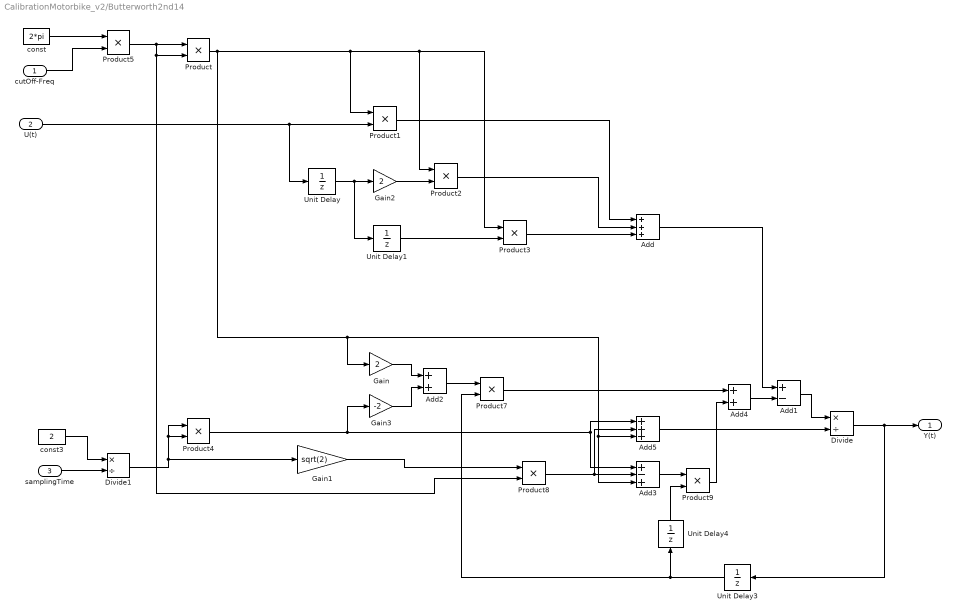
== system CalibrationMotorbike_v2/Butterworth2nd14 ==
  cutOff-Freq : Inport
  U(t) : Inport  Port=2
  samplingTime : Inport  Port=3
  Add : Sum  Inputs=+++
  Add1 : Sum  Inputs=+-
  Add2 : Sum
  Add3 : Sum  Inputs=+-+
  Add4 : Sum
  Add5 : Sum  Inputs=+++
  Divide : Product  Inputs=*/
  Divide1 : Product  Inputs=*/
  Gain : Gain  Gain=2
  Gain1 : Gain  Gain=sqrt(2)
  Gain2 : Gain  Gain=2
  Gain3 : Gain  Gain=-2
  Product{,1..5,7..9} (9 alike) : Product  RndMeth=Zero
  Unit Delay{,1,3..4} (4 alike) : UnitDelay  SampleTime=-1  HasFrameUpgradeWarning=on
  const : Constant  Value=2*pi
  const3 : Constant  Value=2
  Y(t) : Outport  VectorParamsAs1DForOutWhenUnconnected=off
  wires:
  U(t)/1 -> Product1/2, Unit Delay/1
  Product/1 -> Product1/1, Product3/1, Product2/1, Gain/1, Add3/3, Add5/3
  Unit Delay/1 -> Unit Delay1/1, Gain2/1
  Unit Delay1/1 -> Product3/2
  Product1/1 -> Add/1
  Product2/1 -> Add/2
  Product3/1 -> Add/3
  Add/1 -> Add1/1
  Divide/1 -> Unit Delay3/1, Y(t)/1
  Product4/1 -> Add3/1, Add5/1, Gain3/1
  Gain/1 -> Add2/1
  Unit Delay3/1 -> Product7/2, Unit Delay4/1
  Add2/1 -> Product7/1
  Gain1/1 -> Product8/1
  Product8/1 -> Add3/2, Add5/2
  Unit Delay4/1 -> Product9/2
  Add3/1 -> Product9/1
  Product9/1 -> Add4/2
  Product7/1 -> Add4/1
  Add4/1 -> Add1/2
  Add1/1 -> Divide/1
  Add5/1 -> Divide/2
  Gain2/1 -> Product2/2
  Gain3/1 -> Add2/2
  Product5/1 -> Product/1, Product/2, Product8/2
  const/1 -> Product5/1
  cutOff-Freq/1 -> Product5/2
  const3/1 -> Divide1/1
  samplingTime/1 -> Divide1/2
  Divide1/1 -> Gain1/1, Product4/2, Product4/1

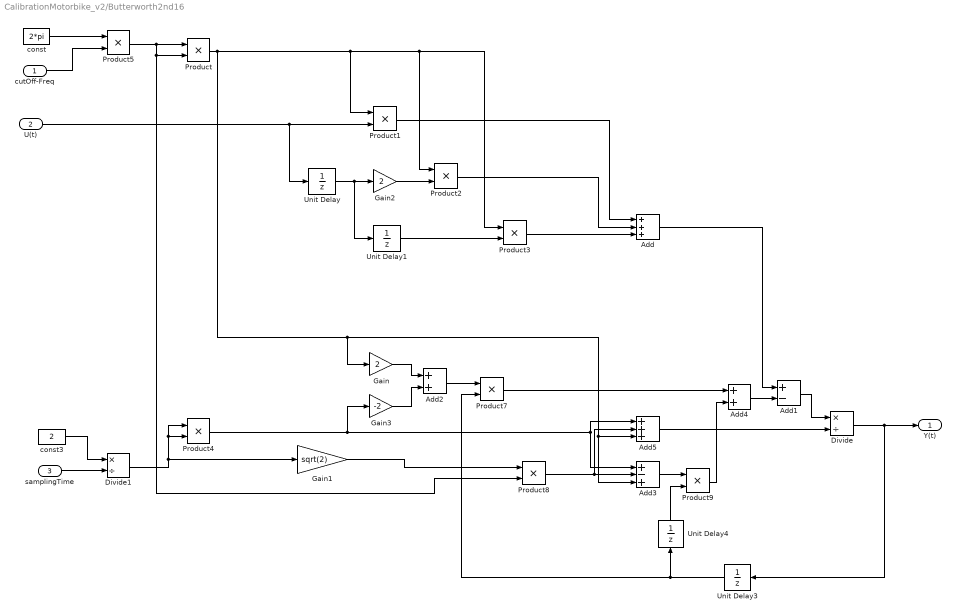
== system CalibrationMotorbike_v2/Butterworth2nd16 ==
  cutOff-Freq : Inport
  U(t) : Inport  Port=2
  samplingTime : Inport  Port=3
  Add : Sum  Inputs=+++
  Add1 : Sum  Inputs=+-
  Add2 : Sum
  Add3 : Sum  Inputs=+-+
  Add4 : Sum
  Add5 : Sum  Inputs=+++
  Divide : Product  Inputs=*/
  Divide1 : Product  Inputs=*/
  Gain : Gain  Gain=2
  Gain1 : Gain  Gain=sqrt(2)
  Gain2 : Gain  Gain=2
  Gain3 : Gain  Gain=-2
  Product{,1..5,7..9} (9 alike) : Product  RndMeth=Zero
  Unit Delay{,1,3..4} (4 alike) : UnitDelay  SampleTime=-1  HasFrameUpgradeWarning=on
  const : Constant  Value=2*pi
  const3 : Constant  Value=2
  Y(t) : Outport  VectorParamsAs1DForOutWhenUnconnected=off
  wires:
  Divide1/1 -> Product4/1, Product4/2, Gain1/1
  samplingTime/1 -> Divide1/2
  const3/1 -> Divide1/1
  cutOff-Freq/1 -> Product5/2
  const/1 -> Product5/1
  Product5/1 -> Product8/2, Product/2, Product/1
  Gain3/1 -> Add2/2
  Gain2/1 -> Product2/2
  Add5/1 -> Divide/2
  Add1/1 -> Divide/1
  Add4/1 -> Add1/2
  Product7/1 -> Add4/1
  Product9/1 -> Add4/2
  Add3/1 -> Product9/1
  Unit Delay4/1 -> Product9/2
  Product8/1 -> Add5/2, Add3/2
  Gain1/1 -> Product8/1
  Add2/1 -> Product7/1
  Unit Delay3/1 -> Unit Delay4/1, Product7/2
  Gain/1 -> Add2/1
  Product4/1 -> Gain3/1, Add5/1, Add3/1
  Divide/1 -> Y(t)/1, Unit Delay3/1
  Add/1 -> Add1/1
  Product3/1 -> Add/3
  Product2/1 -> Add/2
  Product1/1 -> Add/1
  Unit Delay1/1 -> Product3/2
  Unit Delay/1 -> Gain2/1, Unit Delay1/1
  Product/1 -> Add5/3, Add3/3, Gain/1, Product2/1, Product3/1, Product1/1
  U(t)/1 -> Unit Delay/1, Product1/2

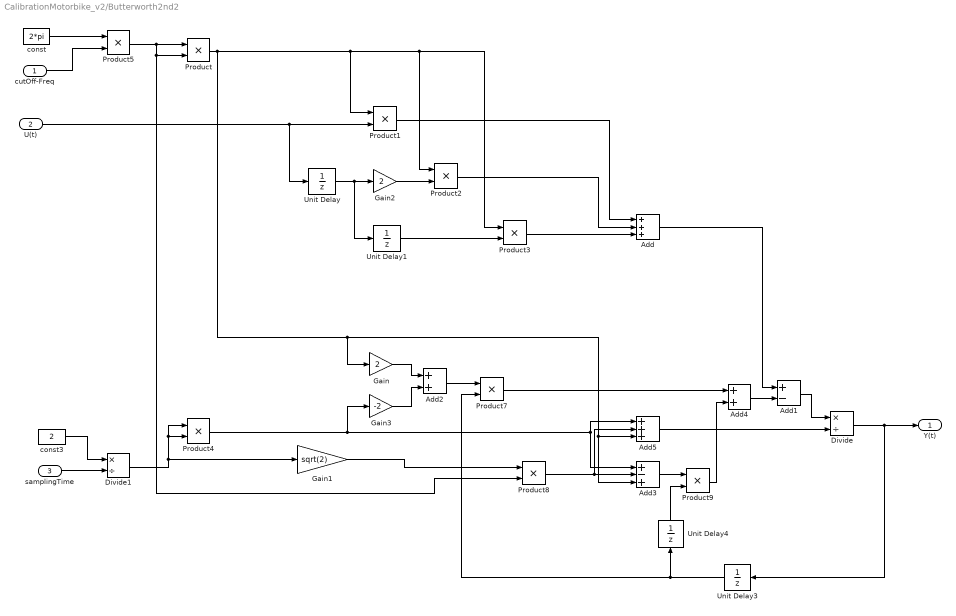
== system CalibrationMotorbike_v2/Butterworth2nd2 ==
  cutOff-Freq : Inport
  U(t) : Inport  Port=2
  samplingTime : Inport  Port=3
  Add : Sum  Inputs=+++
  Add1 : Sum  Inputs=+-
  Add2 : Sum
  Add3 : Sum  Inputs=+-+
  Add4 : Sum
  Add5 : Sum  Inputs=+++
  Divide : Product  Inputs=*/
  Divide1 : Product  Inputs=*/
  Gain : Gain  Gain=2
  Gain1 : Gain  Gain=sqrt(2)
  Gain2 : Gain  Gain=2
  Gain3 : Gain  Gain=-2
  Product{,1..5,7..9} (9 alike) : Product  RndMeth=Zero
  Unit Delay{,1,3..4} (4 alike) : UnitDelay  SampleTime=-1  HasFrameUpgradeWarning=on
  const : Constant  Value=2*pi
  const3 : Constant  Value=2
  Y(t) : Outport  VectorParamsAs1DForOutWhenUnconnected=off
  wires:
  Divide1/1 -> Product4/1, Product4/2, Gain1/1
  samplingTime/1 -> Divide1/2
  const3/1 -> Divide1/1
  cutOff-Freq/1 -> Product5/2
  const/1 -> Product5/1
  Product5/1 -> Product8/2, Product/2, Product/1
  Gain3/1 -> Add2/2
  Gain2/1 -> Product2/2
  Add5/1 -> Divide/2
  Add1/1 -> Divide/1
  Add4/1 -> Add1/2
  Product7/1 -> Add4/1
  Product9/1 -> Add4/2
  Add3/1 -> Product9/1
  Unit Delay4/1 -> Product9/2
  Product8/1 -> Add5/2, Add3/2
  Gain1/1 -> Product8/1
  Add2/1 -> Product7/1
  Unit Delay3/1 -> Unit Delay4/1, Product7/2
  Gain/1 -> Add2/1
  Product4/1 -> Gain3/1, Add5/1, Add3/1
  Divide/1 -> Y(t)/1, Unit Delay3/1
  Add/1 -> Add1/1
  Product3/1 -> Add/3
  Product2/1 -> Add/2
  Product1/1 -> Add/1
  Unit Delay1/1 -> Product3/2
  Unit Delay/1 -> Gain2/1, Unit Delay1/1
  Product/1 -> Add5/3, Add3/3, Gain/1, Product2/1, Product3/1, Product1/1
  U(t)/1 -> Unit Delay/1, Product1/2

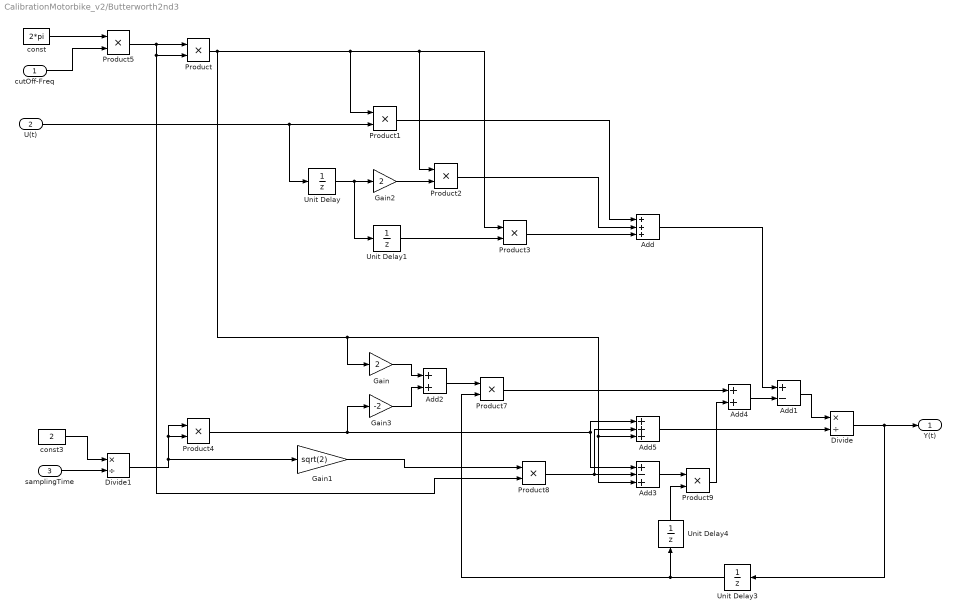
== system CalibrationMotorbike_v2/Butterworth2nd3 ==
  cutOff-Freq : Inport
  U(t) : Inport  Port=2
  samplingTime : Inport  Port=3
  Add : Sum  Inputs=+++
  Add1 : Sum  Inputs=+-
  Add2 : Sum
  Add3 : Sum  Inputs=+-+
  Add4 : Sum
  Add5 : Sum  Inputs=+++
  Divide : Product  Inputs=*/
  Divide1 : Product  Inputs=*/
  Gain : Gain  Gain=2
  Gain1 : Gain  Gain=sqrt(2)
  Gain2 : Gain  Gain=2
  Gain3 : Gain  Gain=-2
  Product{,1..5,7..9} (9 alike) : Product  RndMeth=Zero
  Unit Delay{,1,3..4} (4 alike) : UnitDelay  SampleTime=-1  HasFrameUpgradeWarning=on
  const : Constant  Value=2*pi
  const3 : Constant  Value=2
  Y(t) : Outport  VectorParamsAs1DForOutWhenUnconnected=off
  wires:
  U(t)/1 -> Product1/2, Unit Delay/1
  Product/1 -> Product1/1, Product3/1, Product2/1, Gain/1, Add3/3, Add5/3
  Unit Delay/1 -> Unit Delay1/1, Gain2/1
  Unit Delay1/1 -> Product3/2
  Product1/1 -> Add/1
  Product2/1 -> Add/2
  Product3/1 -> Add/3
  Add/1 -> Add1/1
  Divide/1 -> Unit Delay3/1, Y(t)/1
  Product4/1 -> Add3/1, Add5/1, Gain3/1
  Gain/1 -> Add2/1
  Unit Delay3/1 -> Product7/2, Unit Delay4/1
  Add2/1 -> Product7/1
  Gain1/1 -> Product8/1
  Product8/1 -> Add3/2, Add5/2
  Unit Delay4/1 -> Product9/2
  Add3/1 -> Product9/1
  Product9/1 -> Add4/2
  Product7/1 -> Add4/1
  Add4/1 -> Add1/2
  Add1/1 -> Divide/1
  Add5/1 -> Divide/2
  Gain2/1 -> Product2/2
  Gain3/1 -> Add2/2
  Product5/1 -> Product/1, Product/2, Product8/2
  const/1 -> Product5/1
  cutOff-Freq/1 -> Product5/2
  const3/1 -> Divide1/1
  samplingTime/1 -> Divide1/2
  Divide1/1 -> Gain1/1, Product4/2, Product4/1

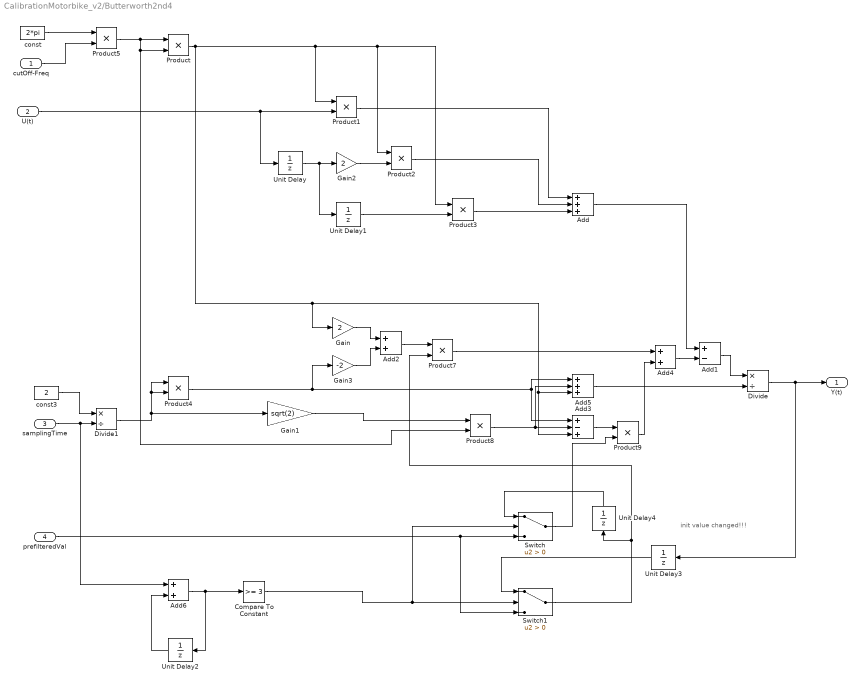
== system CalibrationMotorbike_v2/Butterworth2nd4 ==
  note: init value changed!!!
  cutOff-Freq : Inport
  U(t) : Inport  Port=2
  samplingTime : Inport  Port=3
  prefilteredVal : Inport  Port=4
  Add : Sum  Inputs=+++
  Add1 : Sum  Inputs=+-
  Add2 : Sum
  Add3 : Sum  Inputs=+-+
  Add4 : Sum
  Add5 : Sum  Inputs=+++
  Add6 : Sum
  Compare To Constant : simulink/Logic and Bit Operations/Compare To Constant  relop=>=  const=3  OutDataTypeStr=boolean
  Divide : Product  Inputs=*/
  Divide1 : Product  Inputs=*/
  Gain : Gain  Gain=2
  Gain1 : Gain  Gain=sqrt(2)
  Gain2 : Gain  Gain=2
  Gain3 : Gain  Gain=-2
  Product{,1..5,7..9} (9 alike) : Product  RndMeth=Zero
  Switch : Switch  Criteria=u2 > Threshold
  Switch1 : Switch  Criteria=u2 > Threshold
  Unit Delay{,1..4} (5 alike) : UnitDelay  SampleTime=-1  HasFrameUpgradeWarning=on
  const : Constant  Value=2*pi
  const3 : Constant  Value=2
  Y(t) : Outport  VectorParamsAs1DForOutWhenUnconnected=off
  wires:
  Divide1/1 -> Product4/1, Product4/2, Gain1/1
  samplingTime/1 -> Add6/1, Divide1/2
  const3/1 -> Divide1/1
  cutOff-Freq/1 -> Product5/2
  const/1 -> Product5/1
  Product5/1 -> Product8/2, Product/2, Product/1
  Gain3/1 -> Add2/2
  Gain2/1 -> Product2/2
  Add5/1 -> Divide/2
  Add1/1 -> Divide/1
  Add4/1 -> Add1/2
  Product7/1 -> Add4/1
  Product9/1 -> Add4/2
  Add3/1 -> Product9/1
  Unit Delay4/1 -> Switch/1
  Product8/1 -> Add5/2, Add3/2
  Gain1/1 -> Product8/1
  Add2/1 -> Product7/1
  Gain/1 -> Add2/1
  Product4/1 -> Gain3/1, Add5/1, Add3/1
  Divide/1 -> Y(t)/1, Unit Delay3/1
  Add/1 -> Add1/1
  Product3/1 -> Add/3
  Product2/1 -> Add/2
  Product1/1 -> Add/1
  Unit Delay1/1 -> Product3/2
  Unit Delay/1 -> Gain2/1, Unit Delay1/1
  Product/1 -> Add5/3, Add3/3, Gain/1, Product2/1, Product3/1, Product1/1
  U(t)/1 -> Unit Delay/1, Product1/2
  prefilteredVal/1 -> Switch1/3, Switch/3
  Switch/1 -> Product9/2
  Unit Delay3/1 -> Switch1/1
  Switch1/1 -> Unit Delay4/1, Product7/2
  Add6/1 -> Compare To Constant/1, Unit Delay2/1
  Unit Delay2/1 -> Add6/2
  Compare To Constant/1 -> Switch/2, Switch1/2

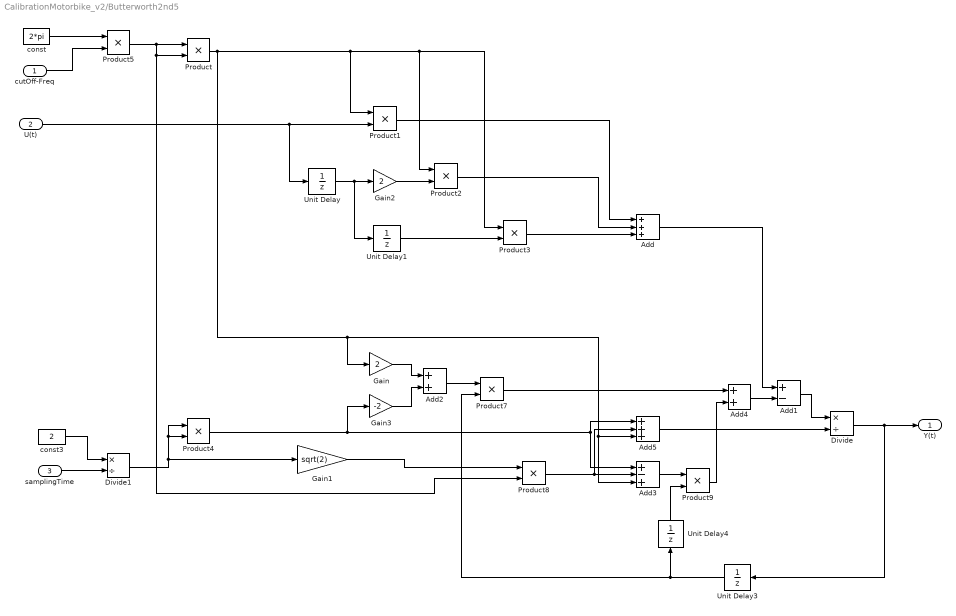
== system CalibrationMotorbike_v2/Butterworth2nd5 ==
  cutOff-Freq : Inport
  U(t) : Inport  Port=2
  samplingTime : Inport  Port=3
  Add : Sum  Inputs=+++
  Add1 : Sum  Inputs=+-
  Add2 : Sum
  Add3 : Sum  Inputs=+-+
  Add4 : Sum
  Add5 : Sum  Inputs=+++
  Divide : Product  Inputs=*/
  Divide1 : Product  Inputs=*/
  Gain : Gain  Gain=2
  Gain1 : Gain  Gain=sqrt(2)
  Gain2 : Gain  Gain=2
  Gain3 : Gain  Gain=-2
  Product{,1..5,7..9} (9 alike) : Product  RndMeth=Zero
  Unit Delay{,1,3..4} (4 alike) : UnitDelay  SampleTime=-1  HasFrameUpgradeWarning=on
  const : Constant  Value=2*pi
  const3 : Constant  Value=2
  Y(t) : Outport  VectorParamsAs1DForOutWhenUnconnected=off
  wires:
  U(t)/1 -> Product1/2, Unit Delay/1
  Product/1 -> Product1/1, Product3/1, Product2/1, Gain/1, Add3/3, Add5/3
  Unit Delay/1 -> Unit Delay1/1, Gain2/1
  Unit Delay1/1 -> Product3/2
  Product1/1 -> Add/1
  Product2/1 -> Add/2
  Product3/1 -> Add/3
  Add/1 -> Add1/1
  Divide/1 -> Unit Delay3/1, Y(t)/1
  Product4/1 -> Add3/1, Add5/1, Gain3/1
  Gain/1 -> Add2/1
  Unit Delay3/1 -> Product7/2, Unit Delay4/1
  Add2/1 -> Product7/1
  Gain1/1 -> Product8/1
  Product8/1 -> Add3/2, Add5/2
  Unit Delay4/1 -> Product9/2
  Add3/1 -> Product9/1
  Product9/1 -> Add4/2
  Product7/1 -> Add4/1
  Add4/1 -> Add1/2
  Add1/1 -> Divide/1
  Add5/1 -> Divide/2
  Gain2/1 -> Product2/2
  Gain3/1 -> Add2/2
  Product5/1 -> Product/1, Product/2, Product8/2
  const/1 -> Product5/1
  cutOff-Freq/1 -> Product5/2
  const3/1 -> Divide1/1
  samplingTime/1 -> Divide1/2
  Divide1/1 -> Gain1/1, Product4/2, Product4/1

== system CalibrationMotorbike_v2/Butterworth2nd6 ==
  cutOff-Freq : Inport
  U(t) : Inport  Port=2
  samplingTime : Inport  Port=3
  Add : Sum  Inputs=+++
  Add1 : Sum  Inputs=+-
  Add2 : Sum
  Add3 : Sum  Inputs=+-+
  Add4 : Sum
  Add5 : Sum  Inputs=+++
  Divide : Product  Inputs=*/
  Divide1 : Product  Inputs=*/
  Gain : Gain  Gain=2
  Gain1 : Gain  Gain=sqrt(2)
  Gain2 : Gain  Gain=2
  Gain3 : Gain  Gain=-2
  Product{,1..5,7..9} (9 alike) : Product  RndMeth=Zero
  Unit Delay{,1,3..4} (4 alike) : UnitDelay  SampleTime=-1  HasFrameUpgradeWarning=on
  const : Constant  Value=2*pi
  const3 : Constant  Value=2
  Y(t) : Outport  VectorParamsAs1DForOutWhenUnconnected=off
  wires:
  Divide1/1 -> Product4/1, Product4/2, Gain1/1
  samplingTime/1 -> Divide1/2
  const3/1 -> Divide1/1
  cutOff-Freq/1 -> Product5/2
  const/1 -> Product5/1
  Product5/1 -> Product8/2, Product/2, Product/1
  Gain3/1 -> Add2/2
  Gain2/1 -> Product2/2
  Add5/1 -> Divide/2
  Add1/1 -> Divide/1
  Add4/1 -> Add1/2
  Product7/1 -> Add4/1
  Product9/1 -> Add4/2
  Add3/1 -> Product9/1
  Unit Delay4/1 -> Product9/2
  Product8/1 -> Add5/2, Add3/2
  Gain1/1 -> Product8/1
  Add2/1 -> Product7/1
  Unit Delay3/1 -> Unit Delay4/1, Product7/2
  Gain/1 -> Add2/1
  Product4/1 -> Gain3/1, Add5/1, Add3/1
  Divide/1 -> Y(t)/1, Unit Delay3/1
  Add/1 -> Add1/1
  Product3/1 -> Add/3
  Product2/1 -> Add/2
  Product1/1 -> Add/1
  Unit Delay1/1 -> Product3/2
  Unit Delay/1 -> Gain2/1, Unit Delay1/1
  Product/1 -> Add5/3, Add3/3, Gain/1, Product2/1, Product3/1, Product1/1
  U(t)/1 -> Unit Delay/1, Product1/2

== system CalibrationMotorbike_v2/Butterworth2nd7 ==
  cutOff-Freq : Inport
  U(t) : Inport  Port=2
  samplingTime : Inport  Port=3
  Add : Sum  Inputs=+++
  Add1 : Sum  Inputs=+-
  Add2 : Sum
  Add3 : Sum  Inputs=+-+
  Add4 : Sum
  Add5 : Sum  Inputs=+++
  Divide : Product  Inputs=*/
  Divide1 : Product  Inputs=*/
  Gain : Gain  Gain=2
  Gain1 : Gain  Gain=sqrt(2)
  Gain2 : Gain  Gain=2
  Gain3 : Gain  Gain=-2
  Product{,1..5,7..9} (9 alike) : Product  RndMeth=Zero
  Unit Delay{,1,3..4} (4 alike) : UnitDelay  SampleTime=-1  HasFrameUpgradeWarning=on
  const : Constant  Value=2*pi
  const3 : Constant  Value=2
  Y(t) : Outport  VectorParamsAs1DForOutWhenUnconnected=off
  wires:
  Divide1/1 -> Product4/1, Product4/2, Gain1/1
  samplingTime/1 -> Divide1/2
  const3/1 -> Divide1/1
  cutOff-Freq/1 -> Product5/2
  const/1 -> Product5/1
  Product5/1 -> Product8/2, Product/2, Product/1
  Gain3/1 -> Add2/2
  Gain2/1 -> Product2/2
  Add5/1 -> Divide/2
  Add1/1 -> Divide/1
  Add4/1 -> Add1/2
  Product7/1 -> Add4/1
  Product9/1 -> Add4/2
  Add3/1 -> Product9/1
  Unit Delay4/1 -> Product9/2
  Product8/1 -> Add5/2, Add3/2
  Gain1/1 -> Product8/1
  Add2/1 -> Product7/1
  Unit Delay3/1 -> Unit Delay4/1, Product7/2
  Gain/1 -> Add2/1
  Product4/1 -> Gain3/1, Add5/1, Add3/1
  Divide/1 -> Y(t)/1, Unit Delay3/1
  Add/1 -> Add1/1
  Product3/1 -> Add/3
  Product2/1 -> Add/2
  Product1/1 -> Add/1
  Unit Delay1/1 -> Product3/2
  Unit Delay/1 -> Gain2/1, Unit Delay1/1
  Product/1 -> Add5/3, Add3/3, Gain/1, Product2/1, Product3/1, Product1/1
  U(t)/1 -> Unit Delay/1, Product1/2

== system CalibrationMotorbike_v2/Butterworth2nd8 ==
  cutOff-Freq : Inport
  U(t) : Inport  Port=2
  samplingTime : Inport  Port=3
  Add : Sum  Inputs=+++
  Add1 : Sum  Inputs=+-
  Add2 : Sum
  Add3 : Sum  Inputs=+-+
  Add4 : Sum
  Add5 : Sum  Inputs=+++
  Divide : Product  Inputs=*/
  Divide1 : Product  Inputs=*/
  Gain : Gain  Gain=2
  Gain1 : Gain  Gain=sqrt(2)
  Gain2 : Gain  Gain=2
  Gain3 : Gain  Gain=-2
  Product{,1..5,7..9} (9 alike) : Product  RndMeth=Zero
  Unit Delay{,1,3..4} (4 alike) : UnitDelay  SampleTime=-1  HasFrameUpgradeWarning=on
  const : Constant  Value=2*pi
  const3 : Constant  Value=2
  Y(t) : Outport  VectorParamsAs1DForOutWhenUnconnected=off
  wires:
  Divide1/1 -> Product4/1, Product4/2, Gain1/1
  samplingTime/1 -> Divide1/2
  const3/1 -> Divide1/1
  cutOff-Freq/1 -> Product5/2
  const/1 -> Product5/1
  Product5/1 -> Product8/2, Product/2, Product/1
  Gain3/1 -> Add2/2
  Gain2/1 -> Product2/2
  Add5/1 -> Divide/2
  Add1/1 -> Divide/1
  Add4/1 -> Add1/2
  Product7/1 -> Add4/1
  Product9/1 -> Add4/2
  Add3/1 -> Product9/1
  Unit Delay4/1 -> Product9/2
  Product8/1 -> Add5/2, Add3/2
  Gain1/1 -> Product8/1
  Add2/1 -> Product7/1
  Unit Delay3/1 -> Unit Delay4/1, Product7/2
  Gain/1 -> Add2/1
  Product4/1 -> Gain3/1, Add5/1, Add3/1
  Divide/1 -> Y(t)/1, Unit Delay3/1
  Add/1 -> Add1/1
  Product3/1 -> Add/3
  Product2/1 -> Add/2
  Product1/1 -> Add/1
  Unit Delay1/1 -> Product3/2
  Unit Delay/1 -> Gain2/1, Unit Delay1/1
  Product/1 -> Add5/3, Add3/3, Gain/1, Product2/1, Product3/1, Product1/1
  U(t)/1 -> Unit Delay/1, Product1/2
